simulink model "my_dom_state_space_2012a"  (R2012a)
settings: Solver=ode45  SolverMode=SingleTasking  StartTime=0.0  StopTime=10000  RelTol=1e-3
undefined symbols (not defined in the file): A, B, C, D, d_T_z, d_T_zew, State_Space_Init, steptime, T_z1, T_zew1
settings Model: CovMetricSettings=dwe  CovHtmlReporting=off  covSaveCumulativeToWorkspaceVar=off  CovSaveSingleToWorkspaceVar=off  CovExternalEMLEnable=on  Creator=johnb  LastModifiedBy=johnb
settings DataIOCC: SaveFormat=StructureWithTime  ReturnWorkspaceOutputs=off
settings OptimizationCC: LifeSpan=inf  SimCompilerOptimization=Off
settings DebuggingCC: FcnCallInpInsideContextMsg=Enable All
settings HardwareCC: ProdWordSize=32  ProdHWDeviceType=Specified
settings SFSimCC: SimUseLocalCustomCode=off
settings RTWCC: RTWUseLocalCustomCode=off  RTWCompilerOptimization=Off
settings GRTTargetCC: CodeReplacementLibrary=C99 (ISO)  CPPClassGenCompliant=off

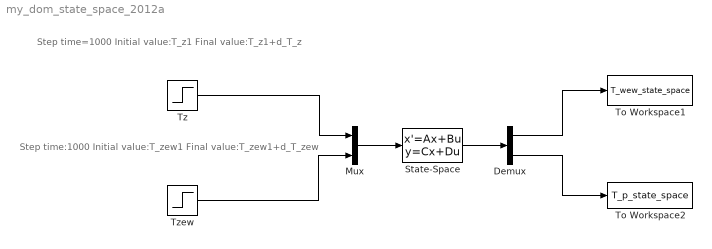
== system my_dom_state_space_2012a ==
  note: Step time=1000
      | Initial value:T_z1
      | Final value:T_z1+d_T_z
  note: Step time:1000
      | Initial value:T_zew1
      | Final value:T_zew1+d_T_zew
  Demux : Demux  Outputs=2
  Mux : Mux  Inputs=2
  State-Space : StateSpace  A=A  B=B  C=C  D=D  X0=State_Space_Init
  To Workspace1 : ToWorkspace  VariableName=T_wew_state_space  SaveFormat=Timeseries  SampleTime=-1
  To Workspace2 : ToWorkspace  VariableName=T_p_state_space  SaveFormat=Timeseries  SampleTime=-1
  Tz : Step  Time=steptime  Before=T_z1  After=T_z1+d_T_z  SampleTime=0
  Tzew : Step  Time=steptime  Before=T_zew1  After=T_zew1+d_T_zew  SampleTime=0
  wires:
  Tz/1 -> Mux/1
  Mux/1 -> State-Space/1
  Demux/1 -> To Workspace1/1
  Demux/2 -> To Workspace2/1
  State-Space/1 -> Demux/1
  Tzew/1 -> Mux/2
